simulink model "inv_pendulum"  (R2025a)
settings: Solver=VariableStepAuto  StartTime=0.0  StopTime=100.0  RelTol=1e-3
values from neighbouring files (symbols this model uses):
  K = lqr(A,B,Q,R)    [CartPuller.m]    (also in Ex12_4.m = acker(A,B,poles); full_state_observer.m = place(A', C', poles_o)'; me23b196_asgn4.m = product_of_pole_magnitudes / product_of_zero_magnitudes)
  x0 = [0;0;pi/3+0.1;0]    [CartPuller.m]    (also in CartPullerODE.m = [0;0;pi+0.1;0]; Controller.m = [1; 0; -1; 0]; JacobCTP.m = [0;0;pi+.1;0]; Observer_4state.m = [-2 0 -10 -1])
settings Model: Creator=abhi  LastModifiedBy=abhi

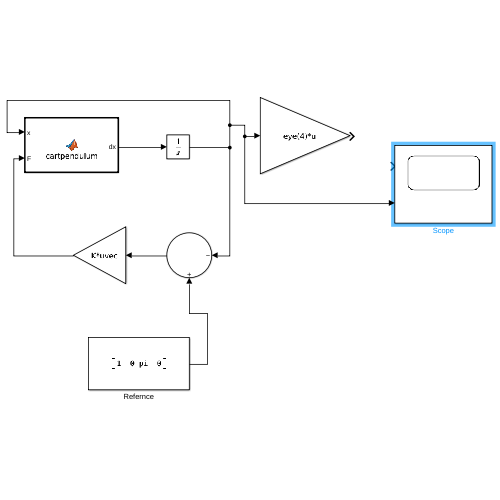
[thumbnail: Simulink's stored preview of the top-level diagram]
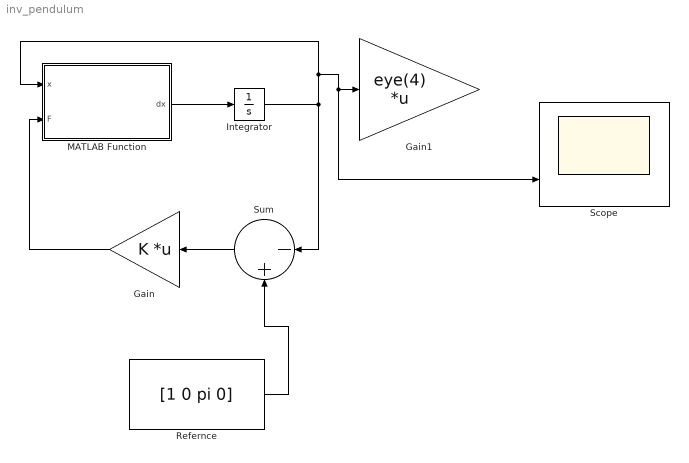
== system inv_pendulum ==
  Gain : Gain  Gain=K  Multiplication=Matrix(K*u) (u vector)
  Gain1 : Gain  Gain=eye(4)  Multiplication=Matrix(K*u)
  Integrator : Integrator  InitialCondition=x0
  MATLAB Function : MATLAB Function  TreatAsAtomicUnit=on
  Refernce : Constant  Value=[1 0 pi 0]
  Scope : Scope  NumInputPorts=2
      settings: ActiveDisplayYMinimum=-5.946533296328667  ActiveDisplayYMaximum=4.34530989824677
  Sum : Sum  Inputs=|-+
  wires:
  Gain/1 -> MATLAB Function/2(F)
  MATLAB Function/1(dx) -> Integrator/1
  Sum/1 -> Gain/1
  Integrator/1 -> Scope/2, Gain1/1, MATLAB Function/1(x), Sum/1
  Refernce/1 -> Sum/2

== matlab function inv_pendulum/MATLAB Function ==
  data: x input; F input; dx output
function dx = cartpendulum(x, F)
    m = 1;
    M = 5;
    l = 2;
    g = 9.81;

    X      = x(1);
    Xdot   = x(2);
    theta  = x(3);
    thetadot = x(4);

    Den = M + m*sin(theta)^2;

    Xddot = (F + m*sin(theta)*(l*thetadot^2 + g*cos(theta))) / Den;

    thetaddot = (-F*cos(theta) - m*l*thetadot^2*cos(theta)*sin(theta) - (M+m)*g*sin(theta)) ...
                / (l*Den);

    dx = [Xdot; Xddot; thetadot; thetaddot];
end
